simulink model "ES90688_p8_2"  (R2018a)
settings: Solver=FixedStepAuto  StartTime=0.0  StopTime=100  FixedStep=1/100  RelTol=1e-3
libraries: fuzblock x1
settings Model: Creator=Diuary  LastModifiedBy=Diuary

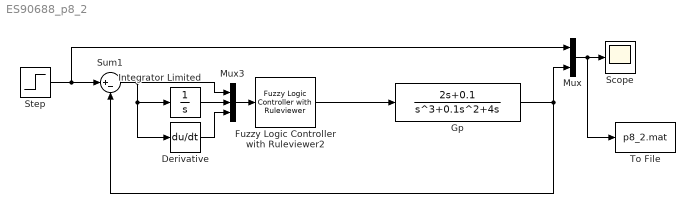
== system ES90688_p8_2 ==
  Derivative : Derivative
  Fuzzy Logic Controller with Ruleviewer2 : fuzblock/Fuzzy Logic  Controller  with Ruleviewer  fismatrix=controle2  Ts=0.1
  Gp : TransferFcn  Numerator=[2 0.1]  Denominator=[1 0.1 4 0]
  Integrator Limited : Integrator  LimitOutput=on  UpperSaturationLimit=1  LowerSaturationLimit=-1
  Mux : Mux  Inputs=2
  Mux3 : Mux  Inputs=3
  Scope : Scope
  Step : Step  SampleTime=0
  Sum1 : Sum  Inputs=|+-
  To File : ToFile  Filename=p8_2.mat  MatrixName=insta  SaveFormat=Timeseries
  wires:
  Mux/1 -> To File/1, Scope/1
  Sum1/1 -> Derivative/1, Integrator Limited/1, Mux3/1
  Gp/1 -> Mux/2, Sum1/2
  Step/1 -> Sum1/1, Mux/1
  Mux3/1 -> Fuzzy Logic Controller with Ruleviewer2/1
  Fuzzy Logic Controller with Ruleviewer2/1 -> Gp/1
  Derivative/1 -> Mux3/3
  Integrator Limited/1 -> Mux3/2
